simulink model "VertMotor_ForceMoment"  (R2025a)
settings: Solver=VariableStepAuto  StartTime=0.0  StopTime=10.0  RelTol=1e-3
settings Model: Creator=19495  LastModifiedBy=19495

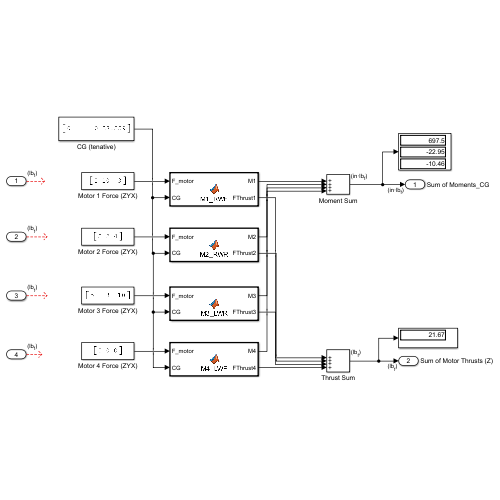
[thumbnail: Simulink's stored preview of the top-level diagram]
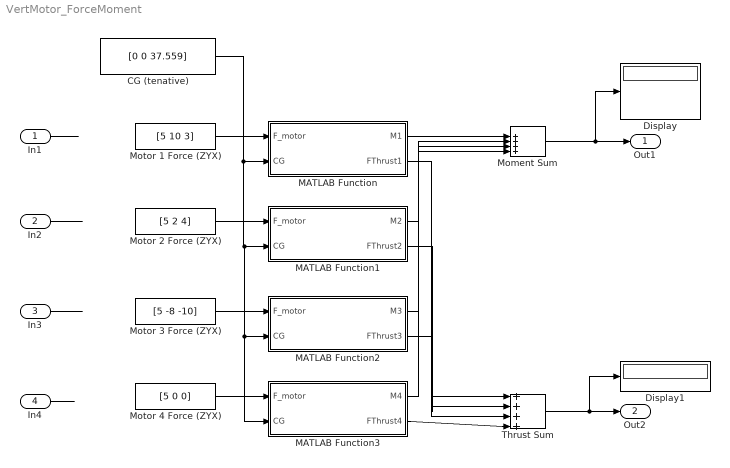
== system VertMotor_ForceMoment ==
  In1 : Inport  Unit=lbf
  In2 : Inport  Port=2  Unit=lbf
  In3 : Inport  Port=3  Unit=lbf
  In4 : Inport  Port=4  Unit=lbf
  CG (tenative) : Constant  Value=[0 0 37.559]  VectorParams1D=off
  Display : Display
  Display1 : Display
  MATLAB Function : MATLAB Function  TreatAsAtomicUnit=on
  MATLAB Function1 : MATLAB Function  TreatAsAtomicUnit=on
  MATLAB Function2 : MATLAB Function  TreatAsAtomicUnit=on
  MATLAB Function3 : MATLAB Function  TreatAsAtomicUnit=on
  Moment Sum : Sum  Inputs=|++++
  Motor 1 Force (ZYX) : Constant  Value=[5 10 3]
  Motor 2 Force (ZYX) : Constant  Value=[5 2 4]
  Motor 3 Force (ZYX) : Constant  Value=[5 -8 -10]
  Motor 4 Force (ZYX) : Constant  Value=[5 0 0]
  Thrust Sum : Sum  Inputs=|++++
  Out1 : Outport  SignalName=Sum of Moments_CG  Unit=in*lbf
  Out2 : Outport  Port=2  SignalName=Sum of Motor Thrusts (Z)  Unit=lbf
  wires:
  Motor 1 Force (ZYX)/1 -> MATLAB Function/1(F_motor)
  Motor 2 Force (ZYX)/1 -> MATLAB Function1/1(F_motor)
  Motor 3 Force (ZYX)/1 -> MATLAB Function2/1(F_motor)
  Motor 4 Force (ZYX)/1 -> MATLAB Function3/1(F_motor)
  Moment Sum/1 -> Out1/1, Display/1
  CG (tenative)/1 -> MATLAB Function3/2(CG), MATLAB Function2/2(CG), MATLAB Function1/2(CG), MATLAB Function/2(CG)
  MATLAB Function/1(M1) -> Moment Sum/1
  MATLAB Function1/1(M2) -> Moment Sum/2
  MATLAB Function2/1(M3) -> Moment Sum/3
  MATLAB Function3/1(M4) -> Moment Sum/4
  MATLAB Function/2(FThrust1) -> Thrust Sum/1
  MATLAB Function1/2(FThrust2) -> Thrust Sum/2
  MATLAB Function2/2(FThrust3) -> Thrust Sum/3
  MATLAB Function3/2(FThrust4) -> Thrust Sum/4
  Thrust Sum/1 -> Out2/1, Display1/1
  In1/1 -> ?
  In3/1 -> ?
  In4/1 -> ?
  In2/1 -> ?

== matlab function VertMotor_ForceMoment/MATLAB Function1 ==
  data: M2 output; F_motor input; FThrust2 output; CG input
function [M2,FThrust2] = M2_RWR(F_motor, CG)
    % Motor positions are from the nose, coordinates from openVSP model (ZYX) 
        % CG is a global variable, dummy value from openVSP currently used 
            %CG = [0 0 37.559];

    tiltangle_deg = 5;                  % Tilt angle of motor 
        theta = deg2rad(tiltangle_deg);
    DCM_x = [cos(theta), sin(theta), 0; % Motor tilt is about the x-axis
             -sin(theta), cos(theta), 0;  % DCM matrix is the same for each side (LW or RW) 
             0, 0, 1];  
 
    F_plane = DCM_x * F_motor; % Motor Force to Plane ZYX
        Fz = abs(F_plane(1, 1)); % Z component of F_dcm for thrust sum 

    M_pos = [0 30 48];
    R = M_pos - CG; % Motor position vector; motor to CG
        
    M = cross(R, F_plane);

M2 = M;
FThrust2 = Fz;

== matlab function VertMotor_ForceMoment/MATLAB Function ==
  data: M1 output; F_motor input; FThrust1 output; CG input
function [M1,FThrust1] = M1_RWF(F_motor, CG)
    % Motor positions are from the nose, coordinates from openVSP model (ZYX) 
        % CG is a global variable, dummy value from openVSP currently used  
            %CG = [0 0 37.559];

    tiltangle_deg = 5;                  % Tilt angle of motor 
        theta = deg2rad(tiltangle_deg);
    DCM_x = [cos(theta), sin(theta), 0; % Motor tilt is about the x-axis
             -sin(theta), cos(theta), 0;
             0, 0, 1];  
 
    F_plane = DCM_x * F_motor; % Motor Force to Plane ZYX
        Fz = abs(F_plane(1, 1)); % Z component of F_dcm for thrust sum 

    M_pos = [0 30 25];
    R = M_pos - CG; % Motor position vector; motor to CG
        
    M = cross(R, F_plane);

M1 = M;
FThrust1 = Fz;

== matlab function VertMotor_ForceMoment/MATLAB Function2 ==
  data: M3 output; F_motor input; FThrust3 output; CG input
function [M3,FThrust3] = M3_LWR(F_motor, CG)
    % Motor positions are from the nose, coordinates from openVSP model (ZYX) 
        % CG is a global variable, dummy value from openVSP currently used 
            %CG = [0 0 37.559];

    tiltangle_deg = 5;                  % Tilt angle of motor 
        theta = deg2rad(tiltangle_deg);
    DCM_x = [cos(theta), -sin(theta), 0; % Motor tilt is about the x-axis
             sin(theta), cos(theta), 0;  % DCM matrix is the same for each side (LW or RW) 
             0, 0, 1];  
 
    F_plane = DCM_x * F_motor; % Motor Force to Plane ZYX
        Fz = abs(F_plane(1, 1)); % Z component of F_dcm for thrust sum 

    M_pos = [0 -30 48];
    R = M_pos - CG; % Motor position vector; motor to CG
        
    M = cross(R, F_plane);

M3 = M;
FThrust3 = Fz;

== matlab function VertMotor_ForceMoment/MATLAB Function3 ==
  data: M4 output; F_motor input; FThrust4 output; CG input
function [M4,FThrust4] = M4_LWF(F_motor, CG)
    % Motor positions are from the nose, coordinates from openVSP model (ZYX) 
        % CG is a global variable, dummy value from openVSP currently used 
            %CG = [0 0 37.559];

    tiltangle_deg = 5;                  % Tilt angle of motor 
        theta = deg2rad(tiltangle_deg);
    DCM_x = [cos(theta), -sin(theta), 0; % Motor tilt is about the x-axis
             sin(theta), cos(theta), 0;  % DCM matrix is the same for each side (LW or RW) 
             0, 0, 1];  
 
    F_plane = DCM_x * F_motor; % Motor Force to Plane ZYX
        Fz = abs(F_plane(1, 1)); % Z component of F_dcm for thrust sum 

    M_pos = [0 -30 25];
    R = M_pos - CG; % Motor position vector; motor to CG
        
    M = cross(R, F_plane);

M4 = M;
FThrust4 = Fz;
